simulink model "Thrust_Deflection_Model"  (R2025b)
settings: Solver=VariableStepAuto  StartTime=0.0  StopTime=10.0  RelTol=1e-3
undefined symbols (not defined in the file or in its folder): params
settings Model: Creator=samue  LastModifiedBy=samue

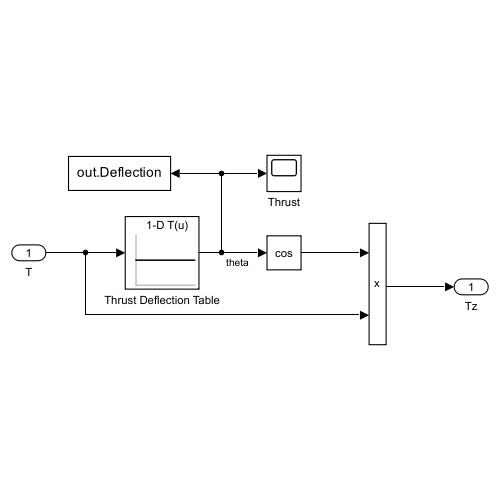
[thumbnail: Simulink's stored preview of the top-level diagram]
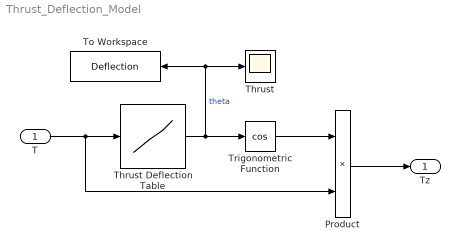
== system Thrust_Deflection_Model ==
  T : Inport
  Product : Product
  Thrust : Scope
  Thrust Deflection Table : Lookup_n-D  NumberOfTableDimensions=1  BreakpointsForDimension1=params.thrust_array_deflection  Table=params.deflection_array  InternalRulePriority=Speed  RndMeth=Simplest
  To Workspace : ToWorkspace  VariableName=Deflection  SaveFormat=Timeseries  SampleTime=-1
  Trigonometric Function : Trigonometry  Operator=cos
  Tz : Outport
  wires:
  Thrust Deflection Table/1 -> Thrust/1, To Workspace/1, Trigonometric Function/1  "theta"
  T/1 -> Product/2, Thrust Deflection Table/1
  Trigonometric Function/1 -> Product/1
  Product/1 -> Tz/1
